simulink model "wind_turbine_simplified"  (R2023b)
settings: Solver=FixedStepAuto  StartTime=0.0  StopTime=50  FixedStep=0.001  RelTol=1e-3
values from neighbouring files (symbols this model uses):
  J_eol = 2*H_tot*P_nom/w_eol_nom^2    (= 921600)    [init_eol_mcc.m]
  omega_tab = v_vent_tab*lambda_opt/R_pal    [init_eol_mcc.m]
  R_pal = 24    [init_eol_mcc.m]
  ro_air = 1.22    [init_eol_mcc.m]
  S_pal = pi*R_pal*R_pal    (= 1809.55736847)    [init_eol_mcc.m]
  w_eol_nom = v_pal_nom/R_pal    (= 3.125)    [init_eol_mcc.m]
undefined symbols (not defined in the file or in its folder): Cp_ref, P_opt_tab2
libraries: ee_lib x2, fl_lib x2, nesl_utility x2, simulink x1
settings Model: Creator=guillaud  LastModifiedBy=gosmann
settings SolverCC: AlgebraicLoopSolver=TrustRegion
settings DataIOCC: LimitDataPoints=on  SaveFormat=Array  SignalLoggingSaveFormat=ModelDataLogs  ReturnWorkspaceOutputs=off
settings OptimizationCC: ExpressionDepthLimit=2147483647  InitFltsAndDblsToZero=on  LifeSpan=inf
settings DebuggingCC: SaveWithParameterizedLinksMsg=none  UnderspecifiedInitializationDetection=Classic  MergeDetectMultiDrivingBlocksExec=none  SignalResolutionControl=TryResolveAllWithWarning  MultiTaskDSMMsg=warning  MultiTaskCondExecSysMsg=none  FcnCallInpInsideContextMsg=warning  UnconnectedInputMsg=warning  UnconnectedOutputMsg=warning  UnconnectedLineMsg=warning  StateNameClashWarn=warning  SFUnexpectedBacktrackingDiag=warning  SFNoUnconditionalDefaultTransitionDiag=warning  SFExecutionAtInitializationDiag=none  ArithmeticOperatorsInVariantConditions=warning
settings HardwareCC: ProdBitPerPointer=32  ProdBitPerSizeT=32  ProdBitPerPtrDiffT=32  ProdLargestAtomicFloat=None  ProdIntDivRoundTo=Undefined  ProdEndianess=Unspecified  ProdWordSize=32  ProdHWDeviceType=32-bit Generic  TargetUnknown=on
settings ModelReferenceCC: EnableRefExpFcnMdlSchedulingChecks=on  PropagateSignalLabelsOutOfModel=off
settings SFSimCC: SimUseLocalCustomCode=off  CustomCodeUndefinedFunction=UseInterfaceOnly
settings RTWCC: RTWUseLocalCustomCode=off  DLArmComputeVersion=19.05
settings CodeAppCC: StateflowObjectComments=on
settings GRTTargetCC: TargetFcnLib=ansi_tfl_tmw.mat  TargetLangStandard=C89/C90 (ANSI)  CombineOutputUpdateFcns=off  GRTInterface=on
settings ConfigComp: CovMetricSettings=dw  CovSaveCumulativeToWorkspaceVar=on  CovSaveSingleToWorkspaceVar=on

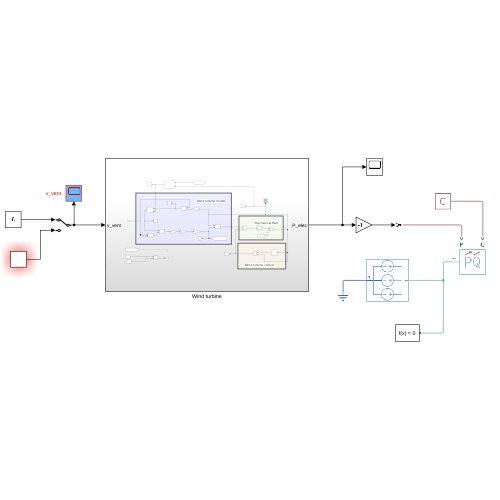
[thumbnail: Simulink's stored preview of the top-level diagram]
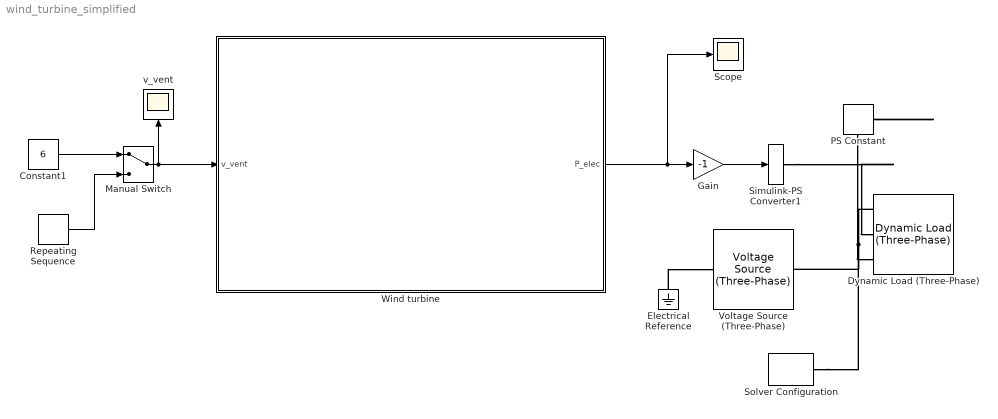
== system wind_turbine_simplified ==
  Constant1 : Constant  Value=6
  Dynamic Load (Three-Phase) : ee_lib/Passive/Dynamic Load (Three-Phase)  port_option=ee.enum.threePhasePort.composite  FRated=60 Hz  Vline_rms_min=100 V  tau=0.01 s  Vline_rms_ini=200 V  Vang_ini=0 deg  gmin=0 S  enable_fault=simscape.enum.onoff.off  fault_action=simscape.enum.assert.action.none  t_fault=1 s  open_conductance=1e-4 S
      settings: InternalSimscapePortConfiguration="{\"Bottom\":[],\"Left\":[{\"id\":\"N\",\"label\":\"~\",\"type\":\"foundation.electrical.three_phase\"}],\"Right\":[],\"Top\":[{\"id\":\"P\",\"label\":\"P\",\"type\":\"input\"},{\"id\":\"Q\",\"label\":\"Q\",\"type\":\"input\"}]}"
  Electrical Reference : fl_lib/Electrical/Electrical Elements/Electrical Reference
  Gain : Gain  Gain=-1
  Manual Switch : ManualSwitch
  PS Constant : fl_lib/Physical Signals/Sources/PS Constant  constant=0
  Repeating Sequence : simulink/Sources/Repeating Sequence  rep_seq_t=t_sim  rep_seq_y=wind_speed6
  Scope : Scope
  Simulink-PS Converter1 : nesl_utility/Simulink-PS Converter  PhysicalDomain=network_engine_domain  SubClassName=ps_input  LeftPortType=input  RightPortType=output  PseudoPeriodic=off  Frequencies=[]  NoiseDistribution=none  NoiseParameters=[]  Unit=1  AffineConversion=off  FilteringAndDerivatives=filter  SimscapeFilterOrder=1  InputFilterTimeConstant=0.001  UdotUserProvided=0
  Solver Configuration : nesl_utility/Solver Configuration  PhysicalDomain=network_engine_domain  SubClassName=solver  LeftPortType=input  RightPortType=generic  Tones=[]  Harmonics=[]  SimulateNoise=off  Profile=off  UseLocalSampling=off  EnableSwitchedLinearOptims=on  FrequencyDomain=off  UseCCode=off  RelTol=0.001  AbsTol=0.001  MinStep=1e-09  ToWorkspace=off  RevertToSquareIcSolve=off  NumHomotopyIterations=100  PhasorMode=off  PhasorModeNumHarmonics=1  ConsistencySolver=NEWTON_XTOL_AFTER_FTOL  IndexReductionMethod=DerivativeReplacement  DoDC=off  ResidualTolerance=1e-09  ConsistencyTolSource=GLOBAL  ConsistencyAbsTol=0.001  ConsistencyRelTol=0.001  ConsistencyTolFactor=0.001  UseLocalSolver=off  LocalSolverChoice=NE_BACKWARD_EULER_ADVANCER  ResolveIndetEquations=on  FunctionEvalNumThread=1  LocalSolverSampleTime=0.001  DoFixedCost=off  MaxNonlinIter=3  MaxModeIter=2  ComputeImpulses=off  ImpulseIterations=2  LinearAlgebra=auto  LinearAlgebraNumThread=0  EquationFormulation=NE_TIME_EF  DelaysMemoryBudget=1024  AutomaticFiltering=on  FilteringTimeConstant=0.001  PartitionStorageMethod=AS_NEEDED  PartitionMemoryBudget=1024  PartitionMethod=ROBUST  MultibodyUseLocalSolver=off  MultibodyLocalSolverChoice=ODE1  MultibodyLocalSolverSampleTime=0.001
  Voltage Source (Three-Phase) : ee_lib/Sources/Voltage Source (Three-Phase)  vline_rms=sqrt(3) * 100 / sqrt(2) V  shift=0 deg  freq=60 Hz  impedance_option=1  SShortCircuit=1e6 A*V  XR=15  R=0.01 Ohm  L=3.97e-4 H  harmonic_option=0  harmonic_orders=[5, 7, 11, 13]  harmonic_ratios=[.1, .1, .1, .1]  G_parasitic=0 1/Ohm  I_specify=off  I_priority=None  I=[0, 0, 0] A  I_nominal_specify=off  I_nominal_unit=A  I_nominal_value=1
  Wind turbine : Subsystem
  "v_vent " : Scope
  wires:
  Constant1/1 -> Manual Switch/1
  Repeating Sequence/1 -> Manual Switch/2
  Manual Switch/1 -> Wind turbine/1(v_vent), "v_vent "/1
  Wind turbine/1(P_elec) -> Gain/1, Scope/1
  Gain/1 -> Simulink-PS Converter1/1
  connections:
  Simulink-PS Converter1/RConn1 -- Dynamic Load (Three-Phase)/LConn2
  PS Constant/RConn1 -- Dynamic Load (Three-Phase)/LConn3
  Dynamic Load (Three-Phase)/LConn1 -- Solver Configuration/RConn1 -- Voltage Source (Three-Phase)/RConn1
  Electrical Reference/LConn1 -- Voltage Source (Three-Phase)/LConn1

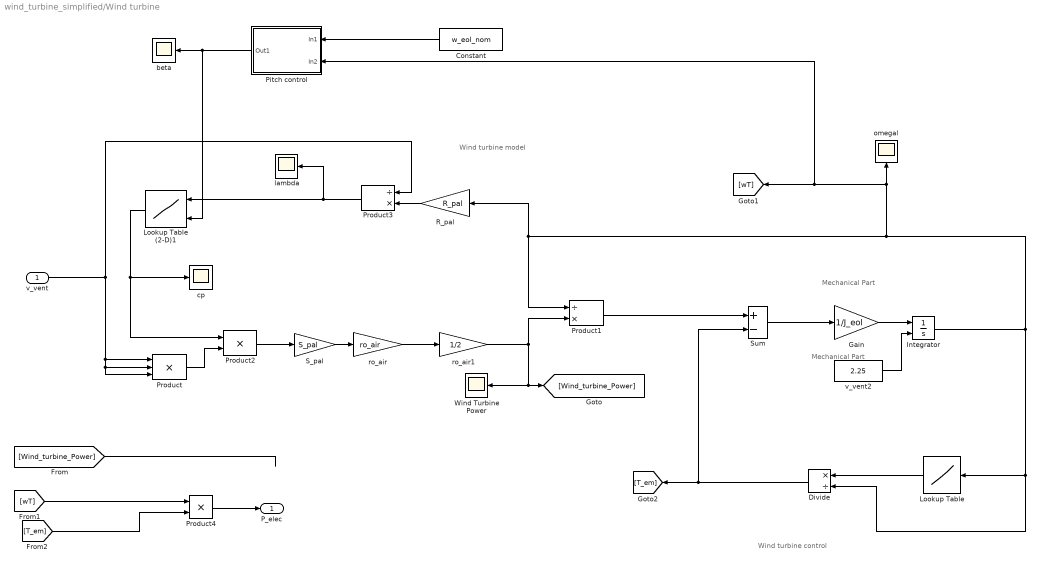
== system wind_turbine_simplified/Wind turbine ==
  note: Wind turbine control
  note: Mechanical Part
  note: Wind turbine model
  note: Mechanical Part
  v_vent : Inport
  Constant : Constant  Value=w_eol_nom
  Divide : Product  Inputs=*/  InputSameDT=on  RndMeth=Zero  OutDataTypeStr=Inherit: Same as first input
  Gain : Gain  Gain=1/J_eol  SaturateOnIntegerOverflow=on  OutDataTypeStr=Inherit: Same as input  ParamDataTypeStr=Inherit: Same as input
  Integrator : Integrator  InitialConditionSource=external
  Lookup Table (2-D)1 : Lookup2D  RowIndex=lambda_ref  ColumnIndex=beta_ref  Table=Cp_ref
  Lookup Table : Lookup  InputValues=omega_tab  Table=P_opt_tab2
  Pitch control : Subsystem
  Product : Product  Inputs=3  InputSameDT=on  RndMeth=Zero  SaturateOnIntegerOverflow=on  OutDataTypeStr=Inherit: Same as first input
  Product1 : Product  Inputs=/*  InputSameDT=on  RndMeth=Zero  SaturateOnIntegerOverflow=on  OutDataTypeStr=Inherit: Same as first input
  Product2 : Product  InputSameDT=on  RndMeth=Zero  SaturateOnIntegerOverflow=on  OutDataTypeStr=Inherit: Same as first input
  Product3 : Product  Inputs=/*  InputSameDT=on  RndMeth=Zero  SaturateOnIntegerOverflow=on  OutDataTypeStr=Inherit: Same as first input
  Product4 : Product
  R_pal : Gain  Gain=R_pal  SaturateOnIntegerOverflow=on  OutDataTypeStr=Inherit: Same as input  ParamDataTypeStr=Inherit: Same as input
  S_pal : Gain  Gain=S_pal  SaturateOnIntegerOverflow=on  OutDataTypeStr=Inherit: Same as input  ParamDataTypeStr=Inherit: Same as input
  Sum : Sum  Inputs=+-  InputSameDT=on  SaturateOnIntegerOverflow=on  OutDataTypeStr=Inherit: Same as first input
  Wind Turbine Power : Scope
  beta : Scope
  cp : Scope
  lambda : Scope
  "omegal  " : Scope
  ro_air : Gain  Gain=ro_air  SaturateOnIntegerOverflow=on  OutDataTypeStr=Inherit: Same as input  ParamDataTypeStr=Inherit: Same as input
  ro_air1 : Gain  Gain=1/2  SaturateOnIntegerOverflow=on  OutDataTypeStr=Inherit: Same as input  ParamDataTypeStr=Inherit: Same as input
  v_vent2 : Constant  Value=2.25
  P_elec : Outport
  wires:
  Sum/1 -> Gain/1
  ro_air1/1 -> Product1/2, Wind Turbine Power/1, [Wind_turbine_Power]
  Product2/1 -> S_pal/1
  R_pal/1 -> Product3/2
  v_vent/1 -> Product3/1, Product/2, Product/3, Product/1
  Product3/1 -> lambda/1, Lookup Table (2-D)1/1
  [wT] -> Product4/1
  Pitch control/1(Out1) -> Lookup Table (2-D)1/2, beta/1
  Constant/1 -> Pitch control/1(In1)
  Product/1 -> Product2/2
  Lookup Table/1 -> Divide/1
  Integrator/1 -> Pitch control/2(In2), [wT], "omegal  "/1, R_pal/1, Product1/1, Lookup Table/1, Divide/2
  S_pal/1 -> ro_air/1
  v_vent2/1 -> Integrator/2
  Lookup Table (2-D)1/1 -> cp/1, Product2/1
  Gain/1 -> Integrator/1
  [T_em] -> Product4/2
  Divide/1 -> Sum/2, [T_em]
  ro_air/1 -> ro_air1/1
  Product1/1 -> Sum/1
  Product4/1 -> P_elec/1
  [Wind_turbine_Power] -> ?

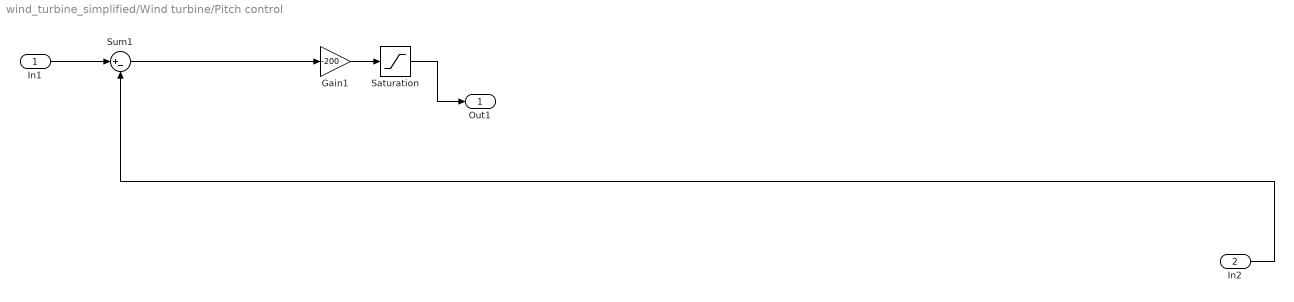
== system wind_turbine_simplified/Wind turbine/Pitch control ==
  In1 : Inport
  In2 : Inport  Port=2
  Gain1 : Gain  Gain=-200
  Saturation : Saturate  UpperLimit=inf  LowerLimit=0
  Sum1 : Sum  Inputs=|+-
  Out1 : Outport
  wires:
  In2/1 -> Sum1/2
  Gain1/1 -> Saturation/1
  Sum1/1 -> Gain1/1
  In1/1 -> Sum1/1
  Saturation/1 -> Out1/1
